simulink model "PDdecouple - 副本 (2)"  (R2021b)
settings: Solver=FixedStepAuto  StartTime=0.0  StopTime=10  FixedStep=1e-3  MaxStep=1e-2  RelTol=1e-5  AbsTol=1e-6
values from neighbouring files (symbols this model uses):
  gravity = [0;0;-9.81]    [parameters.m]
  Inertia = [5.5*10^(-7) 0 0;0 5.5*10^(-7) 0;0 0 11*10^(-7)]    [parameters.m]
  kd = 10    [parameters.m]
  kp = 10    [parameters.m]
  kq = 2500    [parameters.m]
  kw = 50    [parameters.m]
  limite_torque = Inertia*[10;10;10]    [parameters.m]
  Lower_Limit_acc = [-maxacc;-maxacc;-9.81]    [parameters.m]
  mass = 0.027    [parameters.m]
  MaxThrust = 60*1e-3*9.81    (= 0.5886)    [parameters.m]
  Upper_Limit_acc = [maxacc;maxacc;20]    [parameters.m]
libraries: simulink x3, Contact_Forces_Lib x2, sharedutil x1, sharedtransform x1
settings Model: Creator=thinkpad  LastModifiedBy=thinkpad

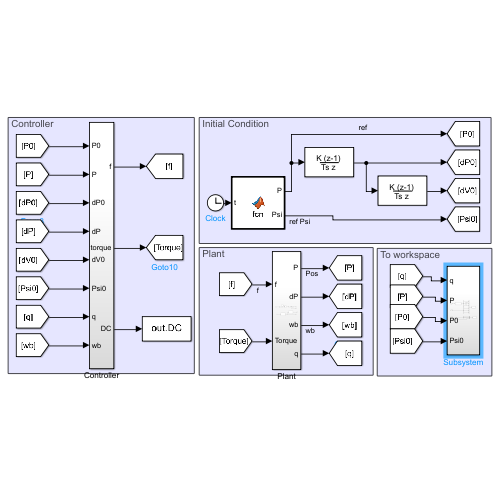
[thumbnail: Simulink's stored preview of the top-level diagram]
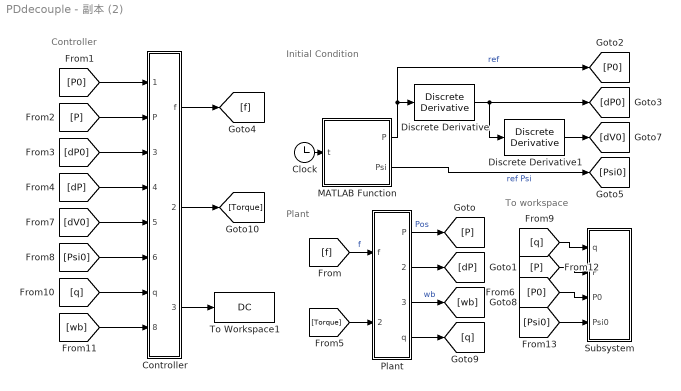
== system PDdecouple - 副本 (2) ==
  note: To workspace
  note: Controller
  note: Initial Condition
  note: Plant
  Clock : Clock
  Controller : Subsystem
  Discrete Derivative : simulink/Discrete/Discrete Derivative  gainval=1.0  ICPrevScaledInput=0.0  OutMin=[]  OutMax=[]  OutDataType=fixdt(1, 16)  OutScaling=2^-10  DoSatur=off
  Discrete Derivative1 : simulink/Discrete/Discrete Derivative  gainval=1.0  ICPrevScaledInput=0.0  OutMin=[]  OutMax=[]  OutDataType=fixdt(1, 16)  OutScaling=2^-10  DoSatur=off
  MATLAB Function : MATLAB Function  TreatAsAtomicUnit=on
  Plant : Subsystem
  Subsystem : Subsystem
  To Workspace1 : ToWorkspace  VariableName=DC  SaveFormat=Timeseries  SampleTime=-1
  wires:
  [Psi0] -> Controller/6(Psi0)
  [wb] -> Controller/8(wb)
  Plant/3(wb) -> [wb]  "wb"
  Plant/2(dP) -> [dP]
  Plant/4(q) -> [q]
  MATLAB Function/1(P) -> [P0], Discrete Derivative/1  "ref"
  MATLAB Function/2(Psi) -> [Psi0]  "ref Psi"
  [Torque] -> Plant/2(Torque)
  [f] -> Plant/1(f)  "f"
  Plant/1(P) -> [P]  "Pos"
  Controller/2(torque) -> [Torque]
  Controller/3(DC) -> To Workspace1/1
  [q] -> Controller/7(q)
  [P0] -> Controller/1(P0)
  [dP] -> Controller/4(dP)
  [P] -> Controller/2(P)
  [dV0] -> Controller/5(dV0)
  [dP0] -> Controller/3(dP0)
  Controller/1(f) -> [f]
  Clock/1 -> MATLAB Function/1(t)
  Discrete Derivative1/1 -> [dV0]
  Discrete Derivative/1 -> [dP0], Discrete Derivative1/1
  [q] -> Subsystem/1(q)
  [P] -> Subsystem/2(P)
  [P0] -> Subsystem/3(P0)
  [Psi0] -> Subsystem/4(Psi0)

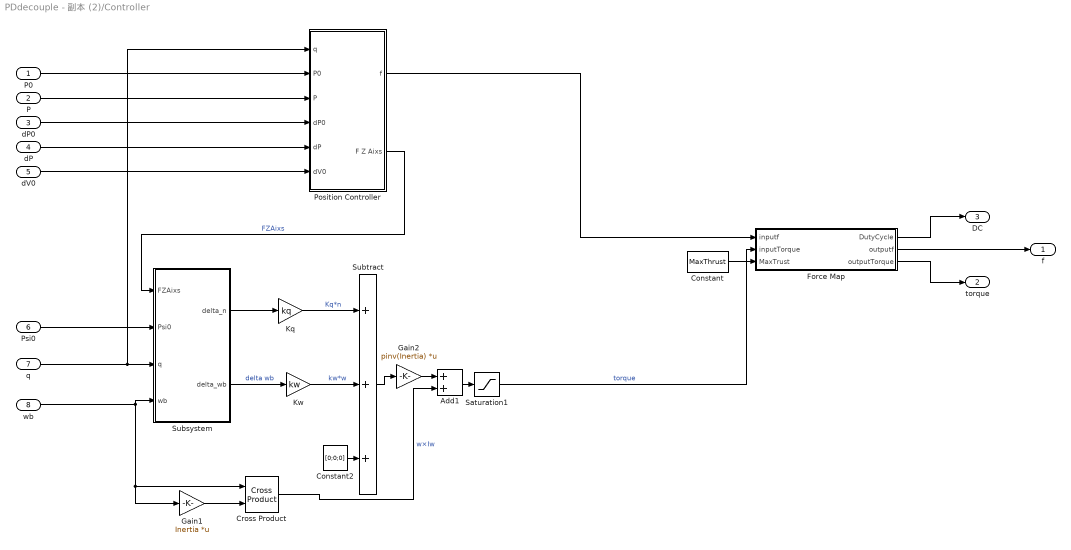
== system PDdecouple - 副本 (2)/Controller ==
  P0 : Inport
  P : Inport  Port=2
  dP0 : Inport  Port=3
  dP : Inport  Port=4
  dV0 : Inport  Port=5
  Psi0 : Inport  Port=6
  q : Inport  Port=7
  wb : Inport  Port=8
  Add1 : Sum
  Constant : Constant  Value=MaxThrust
  Constant2 : Constant  Value=[0;0;0]
  Cross Product : Contact_Forces_Lib/Math/Cross Product  SystemSampleTime=-1  VariantActivationTime=update diagram  Latency=0  AutoFrameSizeCalculation=off
      settings: SourceProductName=Simscape Multibody Contact Forces Library
  Force Map : MATLAB Function  TreatAsAtomicUnit=on
  Gain1 : Gain  Gain=Inertia  Multiplication=Matrix(K*u)
  Gain2 : Gain  Gain=pinv(Inertia)  Multiplication=Matrix(K*u)
  Kq : Gain  Gain=kq
  Kw : Gain  Gain=kw
  Position Controller : Subsystem
  Saturation1 : Saturate  UpperLimit=limite_torque  LowerLimit=-limite_torque
  Subsystem : Subsystem
  Subtract : Sum  Inputs=+++
  f : Outport
  torque : Outport  Port=2
  DC : Outport  Port=3
  wires:
  Kw/1 -> Subtract/2  "kw*w"
  Subsystem/1(delta_n) -> Kq/1
  Subtract/1 -> Gain2/1
  wb/1 -> Cross Product/1, Gain1/1, Subsystem/4(wb)
  q/1 -> Position Controller/1(q), Subsystem/3(q)
  Cross Product/1 -> Add1/2  "w×Iw"
  Subsystem/2(delta_wb) -> Kw/1  "delta wb"
  Gain1/1 -> Cross Product/2
  Constant2/1 -> Subtract/3
  Add1/1 -> Saturation1/1
  Gain2/1 -> Add1/1
  P/1 -> Position Controller/3(P)
  Kq/1 -> Subtract/1  "Kq*n"
  P0/1 -> Position Controller/2(P0)
  Position Controller/2(F Z Aixs) -> Subsystem/1(FZAixs)  "FZAixs"
  Psi0/1 -> Subsystem/2(Psi0)
  dV0/1 -> Position Controller/6(dV0)
  dP0/1 -> Position Controller/4(dP0)
  dP/1 -> Position Controller/5(dP)
  Constant/1 -> Force Map/3(MaxTrust)
  Saturation1/1 -> Force Map/2(inputTorque)  "torque"
  Force Map/2(outputf) -> f/1
  Force Map/3(outputTorque) -> torque/1
  Force Map/1(DutyCycle) -> DC/1
  Position Controller/1(f) -> Force Map/1(inputf)

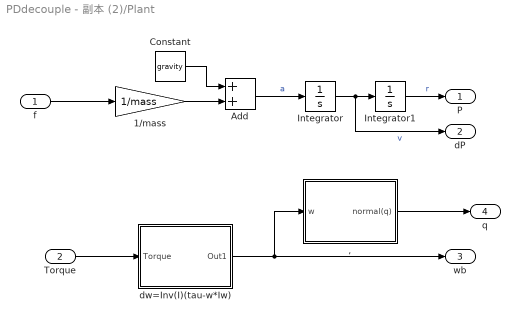
== system PDdecouple - 副本 (2)/Plant ==
  f : Inport
  Torque : Inport  Port=2  PortDimensions=3
  , : Subsystem
  1/mass : Gain  Gain=1/mass
  Add : Sum
  Constant : Constant  Value=gravity
  Integrator : Integrator  InitialCondition=[0;0;0]
  Integrator1 : Integrator  InitialCondition=[0;0;0]
  dw=Inv(I)(tau-w*Iw) : Subsystem
  P : Outport
  dP : Outport  Port=2
  wb : Outport  Port=3
  q : Outport  Port=4
  wires:
  Integrator1/1 -> P/1  "r"
  Constant/1 -> Add/1
  Integrator/1 -> Integrator1/1, dP/1  "v"
  1/mass/1 -> Add/2
  Add/1 -> Integrator/1  "a"
  dw=Inv(I)(tau-w*Iw)/1(Out1) -> wb/1, ,/1(w)
  Torque/1 -> dw=Inv(I)(tau-w*Iw)/1(Torque)
  f/1 -> 1/mass/1
  ,/1(normal(q)) -> q/1

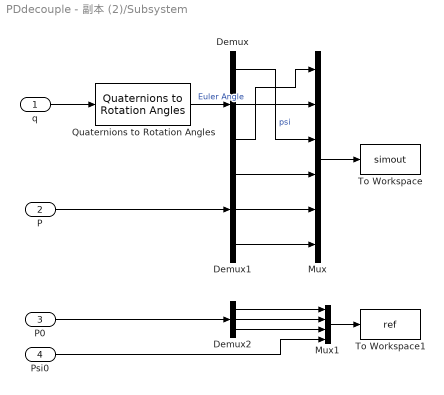
== system PDdecouple - 副本 (2)/Subsystem ==
  q : Inport
  P : Inport  Port=2
  P0 : Inport  Port=3
  Psi0 : Inport  Port=4
  Demux : Demux  Outputs=3
  Demux1 : Demux  Outputs=3
  Demux2 : Demux  Outputs=3
  Mux : Mux  Inputs=6
  Mux1 : Mux
  Quaternions to Rotation Angles : sharedtransform/Quaternions to Rotation Angles  rotationOrder=ZYX  aMode=aMode
      settings: SourceProductBaseCode=AE,PW,DR,MT,UV,VE
  To Workspace : ToWorkspace  VariableName=simout  SampleTime=-1
      settings: Save2DSignal=2-D array (concatenate along first dimension)
  To Workspace1 : ToWorkspace  VariableName=ref  SampleTime=-1
      settings: Save2DSignal=2-D array (concatenate along first dimension)
  wires:
  Demux/1 -> Mux/3  "psi"
  Demux1/3 -> Mux/6
  Mux/1 -> To Workspace/1
  Demux/2 -> Mux/2
  Demux1/2 -> Mux/5
  Demux1/1 -> Mux/4
  Demux/3 -> Mux/1
  Quaternions to Rotation Angles/1 -> Demux/1  "Euler Angle"
  q/1 -> Quaternions to Rotation Angles/1
  P/1 -> Demux1/1
  P0/1 -> Demux2/1
  Demux2/1 -> Mux1/1
  Demux2/2 -> Mux1/2
  Demux2/3 -> Mux1/3
  Psi0/1 -> Mux1/4
  Mux1/1 -> To Workspace1/1

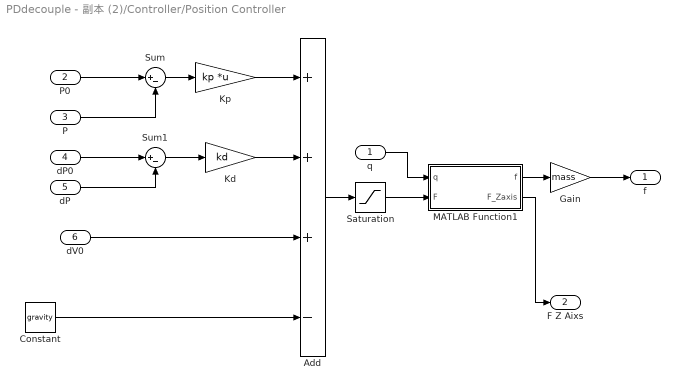
== system PDdecouple - 副本 (2)/Controller/Position Controller ==
  q : Inport
  P0 : Inport  Port=2
  P : Inport  Port=3
  dP0 : Inport  Port=4
  dP : Inport  Port=5
  dV0 : Inport  Port=6
  Add : Sum  Inputs=+++-
  Constant : Constant  Value=gravity
  Gain : Gain  Gain=mass
  Kd : Gain  Gain=kd
  Kp : Gain  Gain=kp  Multiplication=Matrix(K*u)
  MATLAB Function1 : MATLAB Function  TreatAsAtomicUnit=on
  Saturation : Saturate  UpperLimit=Upper_Limit_acc  LowerLimit=Lower_Limit_acc
  Sum : Sum  Inputs=|+-
  Sum1 : Sum  Inputs=|+-
  f : Outport
  F Z Aixs : Outport  Port=2
  wires:
  P/1 -> Sum/2
  Kp/1 -> Add/1
  dP/1 -> Sum1/2
  Sum/1 -> Kp/1
  Sum1/1 -> Kd/1
  Kd/1 -> Add/2
  q/1 -> MATLAB Function1/1(q)
  dP0/1 -> Sum1/1
  dV0/1 -> Add/3
  P0/1 -> Sum/1
  Gain/1 -> f/1
  Add/1 -> Saturation/1
  Saturation/1 -> MATLAB Function1/2(F)
  MATLAB Function1/2(F_Zaxis) -> F Z Aixs/1
  Constant/1 -> Add/4
  MATLAB Function1/1(f) -> Gain/1

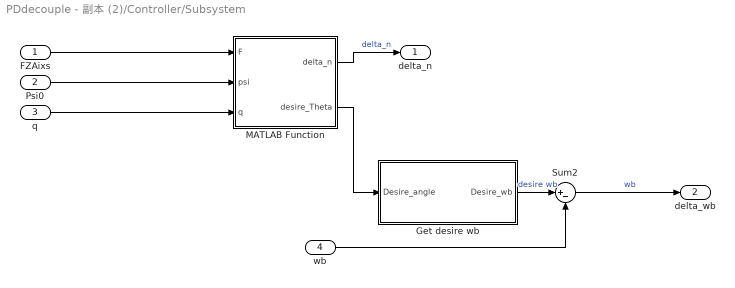
== system PDdecouple - 副本 (2)/Controller/Subsystem ==
  FZAixs : Inport
  Psi0 : Inport  Port=2
  q : Inport  Port=3
  wb : Inport  Port=4
  Get desire wb : Subsystem
  MATLAB Function : MATLAB Function  TreatAsAtomicUnit=on
  Sum2 : Sum  Inputs=|+-
  delta_n : Outport
  delta_wb : Outport  Port=2
  wires:
  wb/1 -> Sum2/2
  Get desire wb/1(Desire_wb) -> Sum2/1  "desire wb"
  q/1 -> MATLAB Function/3(q)
  MATLAB Function/1(delta_n) -> delta_n/1  "delta_n"
  Psi0/1 -> MATLAB Function/2(psi)
  FZAixs/1 -> MATLAB Function/1(F)
  MATLAB Function/2(desire_Theta) -> Get desire wb/1(Desire_angle)
  Sum2/1 -> delta_wb/1  "wb"

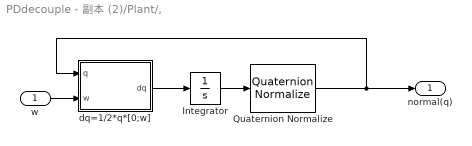
== system PDdecouple - 副本 (2)/Plant/, ==
  w : Inport
  Integrator : Integrator  InitialCondition=[1;0;0;0]
  Quaternion Normalize : sharedutil/Quaternion Normalize  aMode=aMode
      settings: SourceProductBaseCode=AE,PW,DR,MT,UV,VE
  dq=1/2*q*[0;w] : MATLAB Function  TreatAsAtomicUnit=on
  normal(q) : Outport
  wires:
  Quaternion Normalize/1 -> dq=1/2*q*[0;w]/1(q), normal(q)/1
  Integrator/1 -> Quaternion Normalize/1
  dq=1/2*q*[0;w]/1(dq) -> Integrator/1
  w/1 -> dq=1/2*q*[0;w]/2(w)

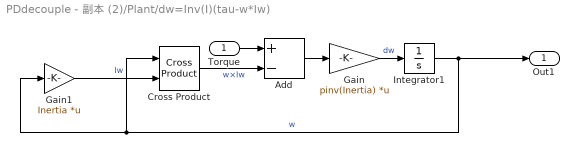
== system PDdecouple - 副本 (2)/Plant/dw=Inv(I)(tau-w*Iw) ==
  Torque : Inport  PortDimensions=3
  Add : Sum  Inputs=+-
  "Cross Product " : Contact_Forces_Lib/Math/Cross Product  SystemSampleTime=-1  VariantActivationTime=update diagram  Latency=0  AutoFrameSizeCalculation=off
      settings: SourceProductName=Simscape Multibody Contact Forces Library
  Gain : Gain  Gain=pinv(Inertia)  Multiplication=Matrix(K*u) (u vector)
  Gain1 : Gain  Gain=Inertia  Multiplication=Matrix(K*u)
  Integrator1 : Integrator  InitialCondition=[0;0;0]
  Out1 : Outport
  wires:
  Gain/1 -> Integrator1/1  "dw"
  "Cross Product "/1 -> Add/2  "w×Iw"
  Integrator1/1 -> Out1/1, Gain1/1, "Cross Product "/1  "w"
  Add/1 -> Gain/1
  Gain1/1 -> "Cross Product "/2  "Iw"
  Torque/1 -> Add/1

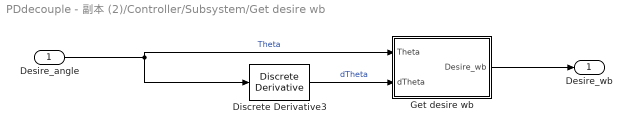
== system PDdecouple - 副本 (2)/Controller/Subsystem/Get desire wb ==
  Desire_angle : Inport
  Discrete Derivative3 : simulink/Discrete/Discrete Derivative  gainval=1.0  ICPrevScaledInput=0.0  OutMin=[]  OutMax=[]  OutDataType=fixdt(1, 16)  OutScaling=2^-10  DoSatur=off
  Get desire wb : MATLAB Function  TreatAsAtomicUnit=on
  Desire_wb : Outport
  wires:
  Discrete Derivative3/1 -> Get desire wb/2(dTheta)  "dTheta"
  Desire_angle/1 -> Get desire wb/1(Theta), Discrete Derivative3/1  "Theta"
  Get desire wb/1(Desire_wb) -> Desire_wb/1

== matlab function PDdecouple - 副本 (2)/Controller/Subsystem/Get desire wb/Get desire wb ==
  data: Theta input size=3; Desire_wb output size=3; dTheta input size=3
function Desire_wb = T_dTheta(Theta, dTheta)
row=Theta(1);
pitch=Theta(2);
yaw=Theta(3);
T=[cos(pitch)*cos(yaw) -sin(yaw) 0;cos(pitch)*sin(yaw) cos(yaw) 0;-sin(pitch) 0 1];
Desire_wb=T*dTheta;
end

== matlab function PDdecouple - 副本 (2)/MATLAB Function ==
  data: t input; P output; Psi output
function [P,Psi] = fcn(t)
x=sin(t)*0.5+0.5;
y=sin(t)*sqrt(0.5);
z=0.5-0.5*exp(-t);

Psi=0;
% P=[1;0;0];
P=[x;0;x];
%Psi=1-exp(-t);
end

== matlab function PDdecouple - 副本 (2)/Plant/,/dq=1//2*q*[0;w] ==
  data: q input; dq output; w input
function dq = fcn(q,w)
dq=1/2*quatmultiply(q.',[0 w.']);
end

== matlab function PDdecouple - 副本 (2)/Controller/Subsystem/MATLAB Function ==
  data: delta_n output size=3; F input size=3; psi input size=1; q input size=4; desire_Theta output
function [delta_n, desire_Theta] = fcn(F, psi, q)
coder.extrinsic('dcm2angle');
coder.extrinsic('dcm2quat');


    u3=F;
    u1=[cos(psi);sin(psi);0];
    u2=cross(u3,u1);
    u2=u2./norm(u2);
    u1=cross(u2,u3);
    R=([u1 u2 u3]).';
    
    q0=zeros(1,4);
    q0=dcm2quat(R);

    desire_Theta=zeros(3,1);
    [desire_Theta(3),desire_Theta(2),desire_Theta(1)]=dcm2angle(R.');



    delta_q=QuatDivide(q0,q.');
    %delta_q=QuatRotation(QuatInv(q),delta_q);
    delta_q=QuatRotation(q,delta_q);
    delta_n=delta_q(2:4);
   
end

== matlab function PDdecouple - 副本 (2)/Controller/Position Controller/MATLAB Function1 ==
  data: q input; f output; F input; F_Zaxis output
function [f,F_Zaxis]= fcn(q,F)
%% calculate the direction of the body

MaxAngle=tan(pi/40);
QuatZAxis=QuatRotation(q,[0;0;0;1]);
if norm(QuatZAxis(2:4))~=0
ZAxis=QuatZAxis(2:4)/norm(QuatZAxis(2:4));
else 
    ZAxis=[0;0;1];
end
% tangentQ=sqrt((ZAxis(1)^2+ZAxis(2)^2)/ZAxis(3)^2);
% alpha=atan(tangent)*sign(ZAxis(1));
% scaleQ=tangentQ/MaxAngle;
%% calculate the direction of the force


% aviod sharp angle of the body
tangentF=sqrt((F(1)^2+F(2)^2)/F(3)^2);
%alpha=atan(1/tangentF)*sign(Fin(1))/pi*1.8;
scaleF=tangentF/MaxAngle;

if scaleF>1
    F(1:2)=F(1:2)./scaleF;
end


%%
%project F to Z axis of the body frame
f=F.'*ZAxis*ZAxis;

if norm(F)==0
    F_Zaxis=[0;0;1];
else
    F_Zaxis=F./norm(F);
end
end

== matlab function PDdecouple - 副本 (2)/Controller/Force Map ==
  data: inputf input size=3; DutyCycle output size=4; inputTorque input size=3; MaxTrust input size=1; outputf output size=3; outputTorque output size=3
function [DutyCycle,outputf,outputTorque] =ForceMap(inputf,inputTorque,MaxTrust)

TransMatrix=[1 1 1 1;
    -0.0046 -0.0046 0.0046 0.0046;
    -0.0046 0.0046 0.0046 -0.0046;
    -0.005964552  0.005964552  -0.005964552  0.005964552];%%%%%%%%%%%%
u=[norm(inputf);inputTorque];

f=TransMatrix\u;
scale1=[1 1 1 1]*f;
for i=1:4
    if f(i)<0
        f(i)=0;
    end
end
scale2=[1 1 1 1]*f;
f=f/scale2*scale1;

if scale1>MaxTrust
    f=f/scale1*MaxTrust;
end

u=TransMatrix*f;
outputf=u(1)*(inputf./norm(inputf)); 
outputTorque=u(2:4);
DutyCycle=Thrust2PWM(f);
end

%%
function dc=Thrust2PWM(f)

% %http://mikehamer.info/assets/papers/Crazyflie%20Modelling.pdf

% a=2.130295*1e-11;
% b=1.032633*1e-6;


a=6.1923723*1e-9;
b=5.467*1e-4;
% c=-0.099-f;
dc=zeros(4,1);


    for i=1:4
        c=-0.099-f(i)/9.81*1e3;
        dc(i)=(-b+sqrt(b^2-4*a*c))/(2*a);
        dc(i)=floor(dc(i))+1;
       
    end
end
%%
